simulink model "MdXX_RspToNetWork"  (R2024b)
settings: Solver=FixedStepDiscrete  StartTime=0.0  StopTime=10.0  FixedStep=0.01  RelTol=1e-3
(part 3 of 3)

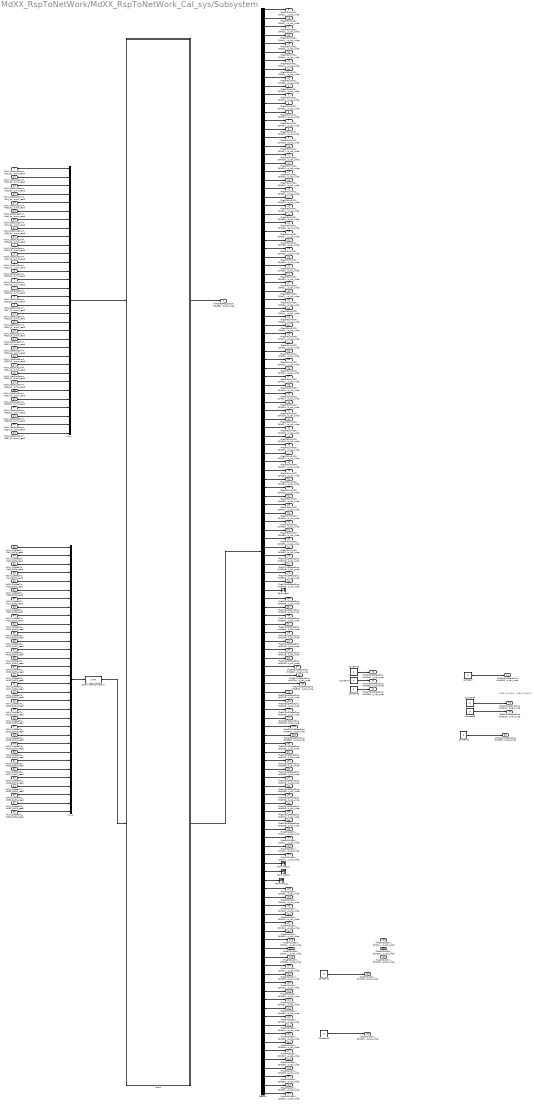
== system MdXX_RspToNetWork/MdXX_RspToNetWork_Cal_sys/Subsystem ==
  note: Md53占用Md18，Md56占用Md25
  MdXX_RspOutComm_Md1_RspOutComm_read : Inport
  MdXX_RspOutComm_Md10_RspOutComm_read : Inport  Port=2
  MdXX_RspOutComm_Md11_RspOutComm_read : Inport  Port=3
  MdXX_RspOutComm_Md12_RspOutComm_read : Inport  Port=4
  MdXX_RspOutComm_Md13_RspOutComm_read : Inport  Port=5
  MdXX_RspOutComm_Md14_RspOutComm_read : Inport  Port=6
  MdXX_RspOutComm_Md15_RspOutComm_read : Inport  Port=7
  MdXX_RspOutComm_Md16_RspOutComm_read : Inport  Port=8
  MdXX_RspOutComm_Md17_RspOutComm_read : Inport  Port=9
  MdXX_RspOutComm_Md18_RspOutComm_read : Inport  Port=10
  MdXX_RspOutComm_Md19_RspOutComm_read : Inport  Port=11
  MdXX_RspOutComm_Md2_RspOutComm_read : Inport  Port=12
  MdXX_RspOutComm_Md20_RspOutComm_read : Inport  Port=13
  MdXX_RspOutComm_Md21_RspOutComm_read : Inport  Port=14
  MdXX_RspOutComm_Md22_RspOutComm_read : Inport  Port=15
  MdXX_RspOutComm_Md23_RspOutComm_read : Inport  Port=16
  MdXX_RspOutComm_Md24_RspOutComm_read : Inport  Port=17
  MdXX_RspOutComm_Md25_RspOutComm_read : Inport  Port=18
  MdXX_RspOutComm_Md26_RspOutComm_read : Inport  Port=19
  MdXX_RspOutComm_Md27_RspOutComm_read : Inport  Port=20
  MdXX_RspOutComm_Md28_RspOutComm_read : Inport  Port=21
  MdXX_RspOutComm_Md29_RspOutComm_read : Inport  Port=22
  MdXX_RspOutComm_Md3_RspOutComm_read : Inport  Port=23
  MdXX_RspOutComm_Md30_RspOutComm_read : Inport  Port=24
  MdXX_RspOutComm_Md31_RspOutComm_read : Inport  Port=25
  MdXX_RspOutComm_Md32_RspOutComm_read : Inport  Port=26
  MdXX_RspOutComm_Md4_RspOutComm_read : Inport  Port=27
  MdXX_RspOutComm_Md5_RspOutComm_read : Inport  Port=28
  MdXX_RspOutComm_Md6_RspOutComm_read : Inport  Port=29
  MdXX_RspOutComm_Md7_RspOutComm_read : Inport  Port=30
  MdXX_RspOutComm_Md8_RspOutComm_read : Inport  Port=31
  MdXX_RspOutComm_Md9_RspOutComm_read : Inport  Port=32
  MdXX_SrcReqTp_Md1_SrcTp_read : Inport  Port=33
  MdXX_SrcReqTp_Md10_SrcTp_read : Inport  Port=34
  MdXX_SrcReqTp_Md11_SrcTp_read : Inport  Port=35
  MdXX_SrcReqTp_Md12_SrcTp_read : Inport  Port=36
  MdXX_SrcReqTp_Md13_SrcTp_read : Inport  Port=37
  MdXX_SrcReqTp_Md14_SrcTp_read : Inport  Port=38
  MdXX_SrcReqTp_Md15_SrcTp_read : Inport  Port=39
  MdXX_SrcReqTp_Md16_SrcTp_read : Inport  Port=40
  MdXX_SrcReqTp_Md17_SrcTp_read : Inport  Port=41
  MdXX_SrcReqTp_Md18_SrcTp_read : Inport  Port=42
  MdXX_SrcReqTp_Md19_SrcTp_read : Inport  Port=43
  MdXX_SrcReqTp_Md2_SrcTp_read : Inport  Port=44
  MdXX_SrcReqTp_Md20_SrcTp_read : Inport  Port=45
  MdXX_SrcReqTp_Md21_SrcTp_read : Inport  Port=46
  MdXX_SrcReqTp_Md22_SrcTp_read : Inport  Port=47
  MdXX_SrcReqTp_Md23_SrcTp_read : Inport  Port=48
  MdXX_SrcReqTp_Md24_SrcTp_read : Inport  Port=49
  MdXX_SrcReqTp_Md25_SrcTp_read : Inport  Port=50
  MdXX_SrcReqTp_Md26_SrcTp_read : Inport  Port=51
  MdXX_SrcReqTp_Md27_SrcTp_read : Inport  Port=52
  MdXX_SrcReqTp_Md28_SrcTp_read : Inport  Port=53
  MdXX_SrcReqTp_Md29_SrcTp_read : Inport  Port=54
  MdXX_SrcReqTp_Md3_SrcTp_read : Inport  Port=55
  MdXX_SrcReqTp_Md30_SrcTp_read : Inport  Port=56
  MdXX_SrcReqTp_Md31_SrcTp_read : Inport  Port=57
  MdXX_SrcReqTp_Md32_SrcTp_read : Inport  Port=58
  MdXX_SrcReqTp_Md4_SrcTp_read : Inport  Port=59
  MdXX_SrcReqTp_Md5_SrcTp_read : Inport  Port=60
  MdXX_SrcReqTp_Md6_SrcTp_read : Inport  Port=61
  MdXX_SrcReqTp_Md7_SrcTp_read : Inport  Port=62
  MdXX_SrcReqTp_Md8_SrcTp_read : Inport  Port=63
  MdXX_SrcReqTp_Md9_SrcTp_read : Inport  Port=64
  Chart : Stateflow chart  TreatAsAtomicUnit=on
  Constant{,1..8} (9 alike) : Constant  Value=0  OutDataTypeStr=uint8
  Data Type Conversion : DataTypeConversion  OutDataTypeStr=uint8  SaturateOnIntegerOverflow=off  RndMeth=Floor
  Demux : Demux  Outputs=128
  Mux : Mux  Inputs=32
  Mux1 : Mux  Inputs=32
  Terminator{,1..3} (4 alike) : Terminator
  IfVeSMStPassCmprtMd_RfCtrl_Sw_RclRspStat_Val_write : Outport  VectorParamsAs1DForOutWhenUnconnected=off
      settings: EnsureOutportIsVirtual=on
  IfVeSMSuHMI2L_StMd1_Rsp_Val_write : Outport  Port=2  VectorParamsAs1DForOutWhenUnconnected=off
      settings: EnsureOutportIsVirtual=on
  IfVeSMSuHMI2L_StMd10_Rsp_Val_write : Outport  Port=3  VectorParamsAs1DForOutWhenUnconnected=off
      settings: EnsureOutportIsVirtual=on
  IfVeSMSuHMI2L_StMd11_Rsp_Val_write : Outport  Port=4  VectorParamsAs1DForOutWhenUnconnected=off
      settings: EnsureOutportIsVirtual=on
  IfVeSMSuHMI2L_StMd12_Rsp_Val_write : Outport  Port=5  VectorParamsAs1DForOutWhenUnconnected=off
      settings: EnsureOutportIsVirtual=on
  IfVeSMSuHMI2L_StMd13_Rsp_Val_write : Outport  Port=6  VectorParamsAs1DForOutWhenUnconnected=off
      settings: EnsureOutportIsVirtual=on
  IfVeSMSuHMI2L_StMd14_Rsp_Val_write : Outport  Port=7  VectorParamsAs1DForOutWhenUnconnected=off
      settings: EnsureOutportIsVirtual=on
  IfVeSMSuHMI2L_StMd15_Rsp_Val_write : Outport  Port=8  VectorParamsAs1DForOutWhenUnconnected=off
      settings: EnsureOutportIsVirtual=on
  IfVeSMSuHMI2L_StMd16_Rsp_Val_write : Outport  Port=9  VectorParamsAs1DForOutWhenUnconnected=off
      settings: EnsureOutportIsVirtual=on
  IfVeSMSuHMI2L_StMd17_Rsp_Val_write : Outport  Port=10  VectorParamsAs1DForOutWhenUnconnected=off
      settings: EnsureOutportIsVirtual=on
  IfVeSMSuHMI2L_StMd18_Rsp_Val_write : Outport  Port=11  VectorParamsAs1DForOutWhenUnconnected=off
      settings: EnsureOutportIsVirtual=on
  IfVeSMSuHMI2L_StMd19_Rsp_Val_write : Outport  Port=12  VectorParamsAs1DForOutWhenUnconnected=off
      settings: EnsureOutportIsVirtual=on
  IfVeSMSuHMI2L_StMd2_Rsp_Val_write : Outport  Port=13  VectorParamsAs1DForOutWhenUnconnected=off
      settings: EnsureOutportIsVirtual=on
  IfVeSMSuHMI2L_StMd20_Rsp_Val_write : Outport  Port=14  VectorParamsAs1DForOutWhenUnconnected=off
      settings: EnsureOutportIsVirtual=on
  IfVeSMSuHMI2L_StMd21_Rsp_Val_write : Outport  Port=15  VectorParamsAs1DForOutWhenUnconnected=off
      settings: EnsureOutportIsVirtual=on
  IfVeSMSuHMI2L_StMd22_Rsp_Val_write : Outport  Port=16  VectorParamsAs1DForOutWhenUnconnected=off
      settings: EnsureOutportIsVirtual=on
  IfVeSMSuHMI2L_StMd23_Rsp_Val_write : Outport  Port=17  VectorParamsAs1DForOutWhenUnconnected=off
      settings: EnsureOutportIsVirtual=on
  IfVeSMSuHMI2L_StMd24_Rsp_Val_write : Outport  Port=18  VectorParamsAs1DForOutWhenUnconnected=off
      settings: EnsureOutportIsVirtual=on
  IfVeSMSuHMI2L_StMd25_Rsp_Val_write : Outport  Port=19  VectorParamsAs1DForOutWhenUnconnected=off
      settings: EnsureOutportIsVirtual=on
  IfVeSMSuHMI2L_StMd26_Rsp_Val_write : Outport  Port=20  VectorParamsAs1DForOutWhenUnconnected=off
      settings: EnsureOutportIsVirtual=on
  IfVeSMSuHMI2L_StMd27_Rsp_Val_write : Outport  Port=21  VectorParamsAs1DForOutWhenUnconnected=off
      settings: EnsureOutportIsVirtual=on
  IfVeSMSuHMI2L_StMd28_Rsp_Val_write : Outport  Port=22  VectorParamsAs1DForOutWhenUnconnected=off
      settings: EnsureOutportIsVirtual=on
  IfVeSMSuHMI2L_StMd29_Rsp_Val_write : Outport  Port=23  VectorParamsAs1DForOutWhenUnconnected=off
      settings: EnsureOutportIsVirtual=on
  IfVeSMSuHMI2L_StMd3_Rsp_Val_write : Outport  Port=24  VectorParamsAs1DForOutWhenUnconnected=off
      settings: EnsureOutportIsVirtual=on
  IfVeSMSuHMI2L_StMd30_Rsp_Val_write : Outport  Port=25  VectorParamsAs1DForOutWhenUnconnected=off
      settings: EnsureOutportIsVirtual=on
  IfVeSMSuHMI2L_StMd31_Rsp_Val_write : Outport  Port=26  VectorParamsAs1DForOutWhenUnconnected=off
      settings: EnsureOutportIsVirtual=on
  IfVeSMSuHMI2L_StMd32_Rsp_Val_write : Outport  Port=27  VectorParamsAs1DForOutWhenUnconnected=off
      settings: EnsureOutportIsVirtual=on
  IfVeSMSuHMI2L_StMd4_Rsp_Val_write : Outport  Port=28  VectorParamsAs1DForOutWhenUnconnected=off
      settings: EnsureOutportIsVirtual=on
  IfVeSMSuHMI2L_StMd5_Rsp_Val_write : Outport  Port=29  VectorParamsAs1DForOutWhenUnconnected=off
      settings: EnsureOutportIsVirtual=on
  IfVeSMSuHMI2L_StMd6_Rsp_Val_write : Outport  Port=30  VectorParamsAs1DForOutWhenUnconnected=off
      settings: EnsureOutportIsVirtual=on
  IfVeSMSuHMI2L_StMd7_Rsp_Val_write : Outport  Port=31  VectorParamsAs1DForOutWhenUnconnected=off
      settings: EnsureOutportIsVirtual=on
  IfVeSMSuHMI2L_StMd8_Rsp_Val_write : Outport  Port=32  VectorParamsAs1DForOutWhenUnconnected=off
      settings: EnsureOutportIsVirtual=on
  IfVeSMSuHMI2L_StMd9_Rsp_Val_write : Outport  Port=33  VectorParamsAs1DForOutWhenUnconnected=off
      settings: EnsureOutportIsVirtual=on
  IfVeSMSuHMI2R_StMd1_Rsp_Val_write : Outport  Port=34  VectorParamsAs1DForOutWhenUnconnected=off
      settings: EnsureOutportIsVirtual=on
  IfVeSMSuHMI2R_StMd10_Rsp_Val_write : Outport  Port=35  VectorParamsAs1DForOutWhenUnconnected=off
      settings: EnsureOutportIsVirtual=on
  IfVeSMSuHMI2R_StMd11_Rsp_Val_write : Outport  Port=36  VectorParamsAs1DForOutWhenUnconnected=off
      settings: EnsureOutportIsVirtual=on
  IfVeSMSuHMI2R_StMd12_Rsp_Val_write : Outport  Port=37  VectorParamsAs1DForOutWhenUnconnected=off
      settings: EnsureOutportIsVirtual=on
  IfVeSMSuHMI2R_StMd13_Rsp_Val_write : Outport  Port=38  VectorParamsAs1DForOutWhenUnconnected=off
      settings: EnsureOutportIsVirtual=on
  IfVeSMSuHMI2R_StMd14_Rsp_Val_write : Outport  Port=39  VectorParamsAs1DForOutWhenUnconnected=off
      settings: EnsureOutportIsVirtual=on
  IfVeSMSuHMI2R_StMd15_Rsp_Val_write : Outport  Port=40  VectorParamsAs1DForOutWhenUnconnected=off
      settings: EnsureOutportIsVirtual=on
  IfVeSMSuHMI2R_StMd16_Rsp_Val_write : Outport  Port=41  VectorParamsAs1DForOutWhenUnconnected=off
      settings: EnsureOutportIsVirtual=on
  IfVeSMSuHMI2R_StMd17_Rsp_Val_write : Outport  Port=42  VectorParamsAs1DForOutWhenUnconnected=off
      settings: EnsureOutportIsVirtual=on
  IfVeSMSuHMI2R_StMd18_Rsp_Val_write : Outport  Port=43  VectorParamsAs1DForOutWhenUnconnected=off
      settings: EnsureOutportIsVirtual=on
  IfVeSMSuHMI2R_StMd19_Rsp_Val_write : Outport  Port=44  VectorParamsAs1DForOutWhenUnconnected=off
      settings: EnsureOutportIsVirtual=on
  IfVeSMSuHMI2R_StMd2_Rsp_Val_write : Outport  Port=45  VectorParamsAs1DForOutWhenUnconnected=off
      settings: EnsureOutportIsVirtual=on
  IfVeSMSuHMI2R_StMd20_Rsp_Val_write : Outport  Port=46  VectorParamsAs1DForOutWhenUnconnected=off
      settings: EnsureOutportIsVirtual=on
  IfVeSMSuHMI2R_StMd21_Rsp_Val_write : Outport  Port=47  VectorParamsAs1DForOutWhenUnconnected=off
      settings: EnsureOutportIsVirtual=on
  IfVeSMSuHMI2R_StMd22_Rsp_Val_write : Outport  Port=48  VectorParamsAs1DForOutWhenUnconnected=off
      settings: EnsureOutportIsVirtual=on
  IfVeSMSuHMI2R_StMd23_Rsp_Val_write : Outport  Port=49  VectorParamsAs1DForOutWhenUnconnected=off
      settings: EnsureOutportIsVirtual=on
  IfVeSMSuHMI2R_StMd24_Rsp_Val_write : Outport  Port=50  VectorParamsAs1DForOutWhenUnconnected=off
      settings: EnsureOutportIsVirtual=on
  IfVeSMSuHMI2R_StMd25_Rsp_Val_write : Outport  Port=51  VectorParamsAs1DForOutWhenUnconnected=off
      settings: EnsureOutportIsVirtual=on
  IfVeSMSuHMI2R_StMd26_Rsp_Val_write : Outport  Port=52  VectorParamsAs1DForOutWhenUnconnected=off
      settings: EnsureOutportIsVirtual=on
  IfVeSMSuHMI2R_StMd27_Rsp_Val_write : Outport  Port=53  VectorParamsAs1DForOutWhenUnconnected=off
      settings: EnsureOutportIsVirtual=on
  IfVeSMSuHMI2R_StMd28_Rsp_Val_write : Outport  Port=54  VectorParamsAs1DForOutWhenUnconnected=off
      settings: EnsureOutportIsVirtual=on
  IfVeSMSuHMI2R_StMd29_Rsp_Val_write : Outport  Port=55  VectorParamsAs1DForOutWhenUnconnected=off
      settings: EnsureOutportIsVirtual=on
  IfVeSMSuHMI2R_StMd3_Rsp_Val_write : Outport  Port=56  VectorParamsAs1DForOutWhenUnconnected=off
      settings: EnsureOutportIsVirtual=on
  IfVeSMSuHMI2R_StMd30_Rsp_Val_write : Outport  Port=57  VectorParamsAs1DForOutWhenUnconnected=off
      settings: EnsureOutportIsVirtual=on
  IfVeSMSuHMI2R_StMd31_Rsp_Val_write : Outport  Port=58  VectorParamsAs1DForOutWhenUnconnected=off
      settings: EnsureOutportIsVirtual=on
  IfVeSMSuHMI2R_StMd32_Rsp_Val_write : Outport  Port=59  VectorParamsAs1DForOutWhenUnconnected=off
      settings: EnsureOutportIsVirtual=on
  IfVeSMSuHMI2R_StMd4_Rsp_Val_write : Outport  Port=60  VectorParamsAs1DForOutWhenUnconnected=off
      settings: EnsureOutportIsVirtual=on
  IfVeSMSuHMI2R_StMd5_Rsp_Val_write : Outport  Port=61  VectorParamsAs1DForOutWhenUnconnected=off
      settings: EnsureOutportIsVirtual=on
  IfVeSMSuHMI2R_StMd6_Rsp_Val_write : Outport  Port=62  VectorParamsAs1DForOutWhenUnconnected=off
      settings: EnsureOutportIsVirtual=on
  IfVeSMSuHMI2R_StMd7_Rsp_Val_write : Outport  Port=63  VectorParamsAs1DForOutWhenUnconnected=off
      settings: EnsureOutportIsVirtual=on
  IfVeSMSuHMI2R_StMd8_Rsp_Val_write : Outport  Port=64  VectorParamsAs1DForOutWhenUnconnected=off
      settings: EnsureOutportIsVirtual=on
  IfVeSMSuHMI2R_StMd9_Rsp_Val_write : Outport  Port=65  VectorParamsAs1DForOutWhenUnconnected=off
      settings: EnsureOutportIsVirtual=on
  IfVeSMSuStPassCmprtMd10RclRspStat_Val_write : Outport  Port=66  VectorParamsAs1DForOutWhenUnconnected=off
      settings: EnsureOutportIsVirtual=on
  IfVeSMSuStPassCmprtMd11RclRspStat_Val_write : Outport  Port=67  VectorParamsAs1DForOutWhenUnconnected=off
      settings: EnsureOutportIsVirtual=on
  IfVeSMSuStPassCmprtMd12RclRspStat_Val_write : Outport  Port=68  VectorParamsAs1DForOutWhenUnconnected=off
      settings: EnsureOutportIsVirtual=on
  IfVeSMSuStPassCmprtMd13RclRspStat_Val_write : Outport  Port=69  VectorParamsAs1DForOutWhenUnconnected=off
      settings: EnsureOutportIsVirtual=on
  IfVeSMSuStPassCmprtMd14RclRspStat_Val_write : Outport  Port=70  VectorParamsAs1DForOutWhenUnconnected=off
      settings: EnsureOutportIsVirtual=on
  IfVeSMSuStPassCmprtMd15RclRspStat_Val_write : Outport  Port=71  VectorParamsAs1DForOutWhenUnconnected=off
      settings: EnsureOutportIsVirtual=on
  IfVeSMSuStPassCmprtMd16RclRspStat_Val_write : Outport  Port=72  VectorParamsAs1DForOutWhenUnconnected=off
      settings: EnsureOutportIsVirtual=on
  IfVeSMSuStPassCmprtMd17RclRspStat_Val_write : Outport  Port=73  VectorParamsAs1DForOutWhenUnconnected=off
      settings: EnsureOutportIsVirtual=on
  IfVeSMSuStPassCmprtMd18RclRspStat_Val_write : Outport  Port=74  VectorParamsAs1DForOutWhenUnconnected=off
      settings: EnsureOutportIsVirtual=on
  IfVeSMSuStPassCmprtMd19RclRspStat_Val_write : Outport  Port=75  VectorParamsAs1DForOutWhenUnconnected=off
      settings: EnsureOutportIsVirtual=on
  IfVeSMSuStPassCmprtMd1RclRspStat_Val_write : Outport  Port=76  VectorParamsAs1DForOutWhenUnconnected=off
      settings: EnsureOutportIsVirtual=on
  IfVeSMSuStPassCmprtMd20RclRspStat_Val_write : Outport  Port=77  VectorParamsAs1DForOutWhenUnconnected=off
      settings: EnsureOutportIsVirtual=on
  IfVeSMSuStPassCmprtMd21RclRspStat_Val_write : Outport  Port=78  VectorParamsAs1DForOutWhenUnconnected=off
      settings: EnsureOutportIsVirtual=on
  IfVeSMSuStPassCmprtMd22RclRspStat_Val_write : Outport  Port=79  VectorParamsAs1DForOutWhenUnconnected=off
      settings: EnsureOutportIsVirtual=on
  IfVeSMSuStPassCmprtMd23RclRspStat_Val_write : Outport  Port=80  VectorParamsAs1DForOutWhenUnconnected=off
      settings: EnsureOutportIsVirtual=on
  IfVeSMSuStPassCmprtMd24RclRspStat_Val_write : Outport  Port=81  VectorParamsAs1DForOutWhenUnconnected=off
      settings: EnsureOutportIsVirtual=on
  IfVeSMSuStPassCmprtMd25RclRspStat_Val_write : Outport  Port=82  VectorParamsAs1DForOutWhenUnconnected=off
      settings: EnsureOutportIsVirtual=on
  IfVeSMSuStPassCmprtMd26RclRspStat_Val_write : Outport  Port=83  VectorParamsAs1DForOutWhenUnconnected=off
      settings: EnsureOutportIsVirtual=on
  IfVeSMSuStPassCmprtMd27RclRspStat_Val_write : Outport  Port=84  VectorParamsAs1DForOutWhenUnconnected=off
      settings: EnsureOutportIsVirtual=on
  IfVeSMSuStPassCmprtMd28RclRspStat_Val_write : Outport  Port=85  VectorParamsAs1DForOutWhenUnconnected=off
      settings: EnsureOutportIsVirtual=on
  IfVeSMSuStPassCmprtMd29RclRspStat_Val_write : Outport  Port=86  VectorParamsAs1DForOutWhenUnconnected=off
      settings: EnsureOutportIsVirtual=on
  IfVeSMSuStPassCmprtMd2RclRspStat_Val_write : Outport  Port=87  VectorParamsAs1DForOutWhenUnconnected=off
      settings: EnsureOutportIsVirtual=on
  IfVeSMSuStPassCmprtMd30RclRspStat_Val_write : Outport  Port=88  VectorParamsAs1DForOutWhenUnconnected=off
      settings: EnsureOutportIsVirtual=on
  IfVeSMSuStPassCmprtMd31RclRspStat_Val_write : Outport  Port=89  VectorParamsAs1DForOutWhenUnconnected=off
      settings: EnsureOutportIsVirtual=on
  IfVeSMSuStPassCmprtMd32RclRspStat_Val_write : Outport  Port=90  VectorParamsAs1DForOutWhenUnconnected=off
      settings: EnsureOutportIsVirtual=on
  IfVeSMSuStPassCmprtMd3RclRspStat_Val_write : Outport  Port=91  VectorParamsAs1DForOutWhenUnconnected=off
      settings: EnsureOutportIsVirtual=on
  IfVeSMSuStPassCmprtMd4RclRspStat_Val_write : Outport  Port=92  VectorParamsAs1DForOutWhenUnconnected=off
      settings: EnsureOutportIsVirtual=on
  IfVeSMSuStPassCmprtMd5RclRspStat_Val_write : Outport  Port=93  VectorParamsAs1DForOutWhenUnconnected=off
      settings: EnsureOutportIsVirtual=on
  IfVeSMSuStPassCmprtMd6RclRspStat_Val_write : Outport  Port=94  VectorParamsAs1DForOutWhenUnconnected=off
      settings: EnsureOutportIsVirtual=on
  IfVeSMSuStPassCmprtMd7RclRspStat_Val_write : Outport  Port=95  VectorParamsAs1DForOutWhenUnconnected=off
      settings: EnsureOutportIsVirtual=on
  IfVeSMSuStPassCmprtMd8RclRspStat_Val_write : Outport  Port=96  VectorParamsAs1DForOutWhenUnconnected=off
      settings: EnsureOutportIsVirtual=on
  IfVeSMSuStPassCmprtMd9RclRspStat_Val_write : Outport  Port=97  VectorParamsAs1DForOutWhenUnconnected=off
      settings: EnsureOutportIsVirtual=on
  IfVeSMSuStSrv_StMd1_Rsp_Val_write : Outport  Port=98  VectorParamsAs1DForOutWhenUnconnected=off
      settings: EnsureOutportIsVirtual=on
  IfVeSMSuStSrv_StMd10_Rsp_Val_write : Outport  Port=99  VectorParamsAs1DForOutWhenUnconnected=off
      settings: EnsureOutportIsVirtual=on
  IfVeSMSuStSrv_StMd11_Rsp_Val_write : Outport  Port=100  VectorParamsAs1DForOutWhenUnconnected=off
      settings: EnsureOutportIsVirtual=on
  IfVeSMSuStSrv_StMd12_Rsp_Val_write : Outport  Port=101  VectorParamsAs1DForOutWhenUnconnected=off
      settings: EnsureOutportIsVirtual=on
  IfVeSMSuStSrv_StMd13_Rsp_Val_write : Outport  Port=102  VectorParamsAs1DForOutWhenUnconnected=off
      settings: EnsureOutportIsVirtual=on
  IfVeSMSuStSrv_StMd14_Rsp_Val_write : Outport  Port=103  VectorParamsAs1DForOutWhenUnconnected=off
      settings: EnsureOutportIsVirtual=on
  IfVeSMSuStSrv_StMd15_Rsp_Val_write : Outport  Port=104  VectorParamsAs1DForOutWhenUnconnected=off
      settings: EnsureOutportIsVirtual=on
  IfVeSMSuStSrv_StMd16_Rsp_Val_write : Outport  Port=105  VectorParamsAs1DForOutWhenUnconnected=off
      settings: EnsureOutportIsVirtual=on
  IfVeSMSuStSrv_StMd17_Rsp_Val_write : Outport  Port=106  VectorParamsAs1DForOutWhenUnconnected=off
      settings: EnsureOutportIsVirtual=on
  IfVeSMSuStSrv_StMd18_Rsp_Val_write : Outport  Port=107  VectorParamsAs1DForOutWhenUnconnected=off
      settings: EnsureOutportIsVirtual=on
  IfVeSMSuStSrv_StMd19_Rsp_Val_write : Outport  Port=108  VectorParamsAs1DForOutWhenUnconnected=off
      settings: EnsureOutportIsVirtual=on
  IfVeSMSuStSrv_StMd2_Rsp_Val_write : Outport  Port=109  VectorParamsAs1DForOutWhenUnconnected=off
      settings: EnsureOutportIsVirtual=on
  IfVeSMSuStSrv_StMd20_Rsp_Val_write : Outport  Port=110  VectorParamsAs1DForOutWhenUnconnected=off
      settings: EnsureOutportIsVirtual=on
  IfVeSMSuStSrv_StMd21_Rsp_Val_write : Outport  Port=111  VectorParamsAs1DForOutWhenUnconnected=off
      settings: EnsureOutportIsVirtual=on
  IfVeSMSuStSrv_StMd22_Rsp_Val_write : Outport  Port=112  VectorParamsAs1DForOutWhenUnconnected=off
      settings: EnsureOutportIsVirtual=on
  IfVeSMSuStSrv_StMd23_Rsp_Val_write : Outport  Port=113  VectorParamsAs1DForOutWhenUnconnected=off
      settings: EnsureOutportIsVirtual=on
  IfVeSMSuStSrv_StMd24_Rsp_Val_write : Outport  Port=114  VectorParamsAs1DForOutWhenUnconnected=off
      settings: EnsureOutportIsVirtual=on
  IfVeSMSuStSrv_StMd25_Rsp_Val_write : Outport  Port=115  VectorParamsAs1DForOutWhenUnconnected=off
      settings: EnsureOutportIsVirtual=on
  IfVeSMSuStSrv_StMd26_Rsp_Val_write : Outport  Port=116  VectorParamsAs1DForOutWhenUnconnected=off
      settings: EnsureOutportIsVirtual=on
  IfVeSMSuStSrv_StMd27_Rsp_Val_write : Outport  Port=117  VectorParamsAs1DForOutWhenUnconnected=off
      settings: EnsureOutportIsVirtual=on
  IfVeSMSuStSrv_StMd28_Rsp_Val_write : Outport  Port=118  VectorParamsAs1DForOutWhenUnconnected=off
      settings: EnsureOutportIsVirtual=on
  IfVeSMSuStSrv_StMd29_Rsp_Val_write : Outport  Port=119  VectorParamsAs1DForOutWhenUnconnected=off
      settings: EnsureOutportIsVirtual=on
  IfVeSMSuStSrv_StMd3_Rsp_Val_write : Outport  Port=120  VectorParamsAs1DForOutWhenUnconnected=off
      settings: EnsureOutportIsVirtual=on
  IfVeSMSuStSrv_StMd30_Rsp_Val_write : Outport  Port=121  VectorParamsAs1DForOutWhenUnconnected=off
      settings: EnsureOutportIsVirtual=on
  IfVeSMSuStSrv_StMd31_Rsp_Val_write : Outport  Port=122  VectorParamsAs1DForOutWhenUnconnected=off
      settings: EnsureOutportIsVirtual=on
  IfVeSMSuStSrv_StMd32_Rsp_Val_write : Outport  Port=123  VectorParamsAs1DForOutWhenUnconnected=off
      settings: EnsureOutportIsVirtual=on
  IfVeSMSuStSrv_StMd4_Rsp_Val_write : Outport  Port=124  VectorParamsAs1DForOutWhenUnconnected=off
      settings: EnsureOutportIsVirtual=on
  IfVeSMSuStSrv_StMd5_Rsp_Val_write : Outport  Port=125  VectorParamsAs1DForOutWhenUnconnected=off
      settings: EnsureOutportIsVirtual=on
  IfVeSMSuStSrv_StMd6_Rsp_Val_write : Outport  Port=126  VectorParamsAs1DForOutWhenUnconnected=off
      settings: EnsureOutportIsVirtual=on
  IfVeSMSuStSrv_StMd7_Rsp_Val_write : Outport  Port=127  VectorParamsAs1DForOutWhenUnconnected=off
      settings: EnsureOutportIsVirtual=on
  IfVeSMSuStSrv_StMd8_Rsp_Val_write : Outport  Port=128  VectorParamsAs1DForOutWhenUnconnected=off
      settings: EnsureOutportIsVirtual=on
  IfVeSMSuStSrv_StMd9_Rsp_Val_write : Outport  Port=129  VectorParamsAs1DForOutWhenUnconnected=off
      settings: EnsureOutportIsVirtual=on
  IfVeSMSuStPassCmprtMd53RclRspStat_Val_write : Outport  Port=130  VectorParamsAs1DForOutWhenUnconnected=off
      settings: EnsureOutportIsVirtual=on
  IfVeSMSuStPassCmprtMd56RclRspStat_Val_write : Outport  Port=131  VectorParamsAs1DForOutWhenUnconnected=off
      settings: EnsureOutportIsVirtual=on
  IfVeSMSuStSrv_StMd53_Rsp_Val_write : Outport  Port=132  VectorParamsAs1DForOutWhenUnconnected=off
      settings: EnsureOutportIsVirtual=on
  IfVeSMSuStSrv_StMd56_Rsp_Val_write : Outport  Port=133  VectorParamsAs1DForOutWhenUnconnected=off
      settings: EnsureOutportIsVirtual=on
  IfVeSMSuStPassCmprtMd57RclRspStat_Val_write : Outport  Port=134  VectorParamsAs1DForOutWhenUnconnected=off
      settings: EnsureOutportIsVirtual=on
  IfVeSMSuStPassCmprtMd58RclRspStat_Val_write : Outport  Port=135  VectorParamsAs1DForOutWhenUnconnected=off
      settings: EnsureOutportIsVirtual=on
  IfVeSMSuStPassCmprtMd61RclRspStat_Val_write : Outport  Port=136  VectorParamsAs1DForOutWhenUnconnected=off
      settings: EnsureOutportIsVirtual=on
  IfVeSMSuStPassCmprtMd62RclRspStat_Val_write : Outport  Port=137  VectorParamsAs1DForOutWhenUnconnected=off
      settings: EnsureOutportIsVirtual=on
  wires:
  MdXX_RspOutComm_Md14_RspOutComm_read/1 -> Mux/14
  MdXX_RspOutComm_Md15_RspOutComm_read/1 -> Mux/15
  MdXX_RspOutComm_Md16_RspOutComm_read/1 -> Mux/16
  MdXX_RspOutComm_Md12_RspOutComm_read/1 -> Mux/12
  MdXX_RspOutComm_Md13_RspOutComm_read/1 -> Mux/13
  MdXX_RspOutComm_Md17_RspOutComm_read/1 -> Mux/17
  MdXX_RspOutComm_Md18_RspOutComm_read/1 -> Mux/18
  MdXX_RspOutComm_Md10_RspOutComm_read/1 -> Mux/10
  MdXX_RspOutComm_Md11_RspOutComm_read/1 -> Mux/11
  MdXX_RspOutComm_Md19_RspOutComm_read/1 -> Mux/19
  MdXX_RspOutComm_Md20_RspOutComm_read/1 -> Mux/20
  MdXX_RspOutComm_Md8_RspOutComm_read/1 -> Mux/8
  MdXX_RspOutComm_Md9_RspOutComm_read/1 -> Mux/9
  MdXX_RspOutComm_Md21_RspOutComm_read/1 -> Mux/21
  MdXX_RspOutComm_Md22_RspOutComm_read/1 -> Mux/22
  MdXX_RspOutComm_Md6_RspOutComm_read/1 -> Mux/6
  MdXX_RspOutComm_Md7_RspOutComm_read/1 -> Mux/7
  MdXX_RspOutComm_Md23_RspOutComm_read/1 -> Mux/23
  MdXX_RspOutComm_Md24_RspOutComm_read/1 -> Mux/24
  MdXX_RspOutComm_Md25_RspOutComm_read/1 -> Mux/25
  MdXX_RspOutComm_Md3_RspOutComm_read/1 -> Mux/3
  MdXX_RspOutComm_Md4_RspOutComm_read/1 -> Mux/4
  MdXX_RspOutComm_Md5_RspOutComm_read/1 -> Mux/5
  MdXX_RspOutComm_Md26_RspOutComm_read/1 -> Mux/26
  MdXX_RspOutComm_Md27_RspOutComm_read/1 -> Mux/27
  MdXX_RspOutComm_Md1_RspOutComm_read/1 -> Mux/1
  MdXX_RspOutComm_Md2_RspOutComm_read/1 -> Mux/2
  MdXX_RspOutComm_Md28_RspOutComm_read/1 -> Mux/28
  MdXX_RspOutComm_Md29_RspOutComm_read/1 -> Mux/29
  MdXX_RspOutComm_Md30_RspOutComm_read/1 -> Mux/30
  MdXX_RspOutComm_Md31_RspOutComm_read/1 -> Mux/31
  MdXX_RspOutComm_Md32_RspOutComm_read/1 -> Mux/32
  Mux/1 -> Chart/1(MdXX_RspOutCommArray)
  MdXX_SrcReqTp_Md10_SrcTp_read/1 -> Mux1/10
  MdXX_SrcReqTp_Md11_SrcTp_read/1 -> Mux1/11
  MdXX_SrcReqTp_Md9_SrcTp_read/1 -> Mux1/9
  MdXX_SrcReqTp_Md12_SrcTp_read/1 -> Mux1/12
  MdXX_SrcReqTp_Md13_SrcTp_read/1 -> Mux1/13
  MdXX_SrcReqTp_Md14_SrcTp_read/1 -> Mux1/14
  MdXX_SrcReqTp_Md6_SrcTp_read/1 -> Mux1/6
  MdXX_SrcReqTp_Md7_SrcTp_read/1 -> Mux1/7
  MdXX_SrcReqTp_Md8_SrcTp_read/1 -> Mux1/8
  MdXX_SrcReqTp_Md15_SrcTp_read/1 -> Mux1/15
  MdXX_SrcReqTp_Md16_SrcTp_read/1 -> Mux1/16
  MdXX_SrcReqTp_Md4_SrcTp_read/1 -> Mux1/4
  MdXX_SrcReqTp_Md5_SrcTp_read/1 -> Mux1/5
  MdXX_SrcReqTp_Md17_SrcTp_read/1 -> Mux1/17
  MdXX_SrcReqTp_Md18_SrcTp_read/1 -> Mux1/18
  MdXX_SrcReqTp_Md19_SrcTp_read/1 -> Mux1/19
  MdXX_SrcReqTp_Md20_SrcTp_read/1 -> Mux1/20
  MdXX_SrcReqTp_Md2_SrcTp_read/1 -> Mux1/2
  MdXX_SrcReqTp_Md3_SrcTp_read/1 -> Mux1/3
  MdXX_SrcReqTp_Md21_SrcTp_read/1 -> Mux1/21
  MdXX_SrcReqTp_Md22_SrcTp_read/1 -> Mux1/22
  MdXX_SrcReqTp_Md23_SrcTp_read/1 -> Mux1/23
  MdXX_SrcReqTp_Md1_SrcTp_read/1 -> Mux1/1
  MdXX_SrcReqTp_Md24_SrcTp_read/1 -> Mux1/24
  MdXX_SrcReqTp_Md25_SrcTp_read/1 -> Mux1/25
  MdXX_SrcReqTp_Md26_SrcTp_read/1 -> Mux1/26
  MdXX_SrcReqTp_Md27_SrcTp_read/1 -> Mux1/27
  MdXX_SrcReqTp_Md28_SrcTp_read/1 -> Mux1/28
  MdXX_SrcReqTp_Md29_SrcTp_read/1 -> Mux1/29
  MdXX_SrcReqTp_Md30_SrcTp_read/1 -> Mux1/30
  MdXX_SrcReqTp_Md31_SrcTp_read/1 -> Mux1/31
  MdXX_SrcReqTp_Md32_SrcTp_read/1 -> Mux1/32
  Mux1/1 -> Data Type Conversion/1
  Data Type Conversion/1 -> Chart/2(MdXX_SrcReqTpArray)
  Chart/1(RfCtrl_Sw_RclRspStat) -> IfVeSMStPassCmprtMd_RfCtrl_Sw_RclRspStat_Val_write/1
  Demux/81 -> IfVeSMSuStPassCmprtMd17RclRspStat_Val_write/1
  Demux/77 -> IfVeSMSuStPassCmprtMd13RclRspStat_Val_write/1
  Demux/83 -> IfVeSMSuStPassCmprtMd19RclRspStat_Val_write/1
  Demux/74 -> IfVeSMSuStPassCmprtMd10RclRspStat_Val_write/1
  Demux/75 -> IfVeSMSuStPassCmprtMd11RclRspStat_Val_write/1
  Demux/76 -> IfVeSMSuStPassCmprtMd12RclRspStat_Val_write/1
  Demux/72 -> IfVeSMSuStPassCmprtMd8RclRspStat_Val_write/1
  Demux/73 -> IfVeSMSuStPassCmprtMd9RclRspStat_Val_write/1
  Demux/84 -> IfVeSMSuStPassCmprtMd20RclRspStat_Val_write/1
  Demux/87 -> IfVeSMSuStPassCmprtMd23RclRspStat_Val_write/1
  Demux/97 -> IfVeSMSuStSrv_StMd1_Rsp_Val_write/1
  Demux/98 -> IfVeSMSuStSrv_StMd2_Rsp_Val_write/1
  Demux/99 -> IfVeSMSuStSrv_StMd3_Rsp_Val_write/1
  Demux/100 -> IfVeSMSuStSrv_StMd4_Rsp_Val_write/1
  Demux/104 -> IfVeSMSuStSrv_StMd8_Rsp_Val_write/1
  Demux/105 -> IfVeSMSuStSrv_StMd9_Rsp_Val_write/1
  Demux/106 -> IfVeSMSuStSrv_StMd10_Rsp_Val_write/1
  Demux/107 -> IfVeSMSuStSrv_StMd11_Rsp_Val_write/1
  Demux/108 -> IfVeSMSuStSrv_StMd12_Rsp_Val_write/1
  Demux/109 -> IfVeSMSuStSrv_StMd13_Rsp_Val_write/1
  Demux/113 -> IfVeSMSuStSrv_StMd17_Rsp_Val_write/1
  Demux/115 -> IfVeSMSuStSrv_StMd19_Rsp_Val_write/1
  Demux/116 -> IfVeSMSuStSrv_StMd20_Rsp_Val_write/1
  Demux/117 -> IfVeSMSuStSrv_StMd21_Rsp_Val_write/1
  Demux/118 -> IfVeSMSuStSrv_StMd22_Rsp_Val_write/1
  Demux/119 -> IfVeSMSuStSrv_StMd23_Rsp_Val_write/1
  Demux/120 -> IfVeSMSuStSrv_StMd24_Rsp_Val_write/1
  Demux/122 -> IfVeSMSuStSrv_StMd26_Rsp_Val_write/1
  Demux/123 -> IfVeSMSuStSrv_StMd27_Rsp_Val_write/1
  Demux/124 -> IfVeSMSuStSrv_StMd28_Rsp_Val_write/1
  Demux/125 -> IfVeSMSuStSrv_StMd29_Rsp_Val_write/1
  Demux/126 -> IfVeSMSuStSrv_StMd30_Rsp_Val_write/1
  Demux/127 -> IfVeSMSuStSrv_StMd31_Rsp_Val_write/1
  Demux/128 -> IfVeSMSuStSrv_StMd32_Rsp_Val_write/1
  Demux/66 -> IfVeSMSuStPassCmprtMd2RclRspStat_Val_write/1
  Demux/67 -> IfVeSMSuStPassCmprtMd3RclRspStat_Val_write/1
  Demux/68 -> IfVeSMSuStPassCmprtMd4RclRspStat_Val_write/1
  Demux/88 -> IfVeSMSuStPassCmprtMd24RclRspStat_Val_write/1
  Demux/90 -> IfVeSMSuStPassCmprtMd26RclRspStat_Val_write/1
  Demux/91 -> IfVeSMSuStPassCmprtMd27RclRspStat_Val_write/1
  Demux/92 -> IfVeSMSuStPassCmprtMd28RclRspStat_Val_write/1
  Demux/65 -> IfVeSMSuStPassCmprtMd1RclRspStat_Val_write/1
  Demux/93 -> IfVeSMSuStPassCmprtMd29RclRspStat_Val_write/1
  Demux/64 -> IfVeSMSuHMI2R_StMd32_Rsp_Val_write/1
  Demux/94 -> IfVeSMSuStPassCmprtMd30RclRspStat_Val_write/1
  Demux/62 -> IfVeSMSuHMI2R_StMd30_Rsp_Val_write/1
  Demux/63 -> IfVeSMSuHMI2R_StMd31_Rsp_Val_write/1
  Demux/95 -> IfVeSMSuStPassCmprtMd31RclRspStat_Val_write/1
  Demux/96 -> IfVeSMSuStPassCmprtMd32RclRspStat_Val_write/1
  Demux/60 -> IfVeSMSuHMI2R_StMd28_Rsp_Val_write/1
  Demux/61 -> IfVeSMSuHMI2R_StMd29_Rsp_Val_write/1
  Demux/57 -> IfVeSMSuHMI2R_StMd25_Rsp_Val_write/1
  Demux/58 -> IfVeSMSuHMI2R_StMd26_Rsp_Val_write/1
  Demux/59 -> IfVeSMSuHMI2R_StMd27_Rsp_Val_write/1
  Demux/55 -> IfVeSMSuHMI2R_StMd23_Rsp_Val_write/1
  Demux/56 -> IfVeSMSuHMI2R_StMd24_Rsp_Val_write/1
  Demux/51 -> IfVeSMSuHMI2R_StMd19_Rsp_Val_write/1
  Demux/52 -> IfVeSMSuHMI2R_StMd20_Rsp_Val_write/1
  Demux/53 -> IfVeSMSuHMI2R_StMd21_Rsp_Val_write/1
  Demux/54 -> IfVeSMSuHMI2R_StMd22_Rsp_Val_write/1
  Demux/48 -> IfVeSMSuHMI2R_StMd16_Rsp_Val_write/1
  Demux/49 -> IfVeSMSuHMI2R_StMd17_Rsp_Val_write/1
  Demux/50 -> IfVeSMSuHMI2R_StMd18_Rsp_Val_write/1
  Demux/46 -> IfVeSMSuHMI2R_StMd14_Rsp_Val_write/1
  Demux/47 -> IfVeSMSuHMI2R_StMd15_Rsp_Val_write/1
  Demux/43 -> IfVeSMSuHMI2R_StMd11_Rsp_Val_write/1
  Demux/44 -> IfVeSMSuHMI2R_StMd12_Rsp_Val_write/1
  Demux/45 -> IfVeSMSuHMI2R_StMd13_Rsp_Val_write/1
  Demux/42 -> IfVeSMSuHMI2R_StMd10_Rsp_Val_write/1
  Demux/40 -> IfVeSMSuHMI2R_StMd8_Rsp_Val_write/1
  Demux/41 -> IfVeSMSuHMI2R_StMd9_Rsp_Val_write/1
  Demux/37 -> IfVeSMSuHMI2R_StMd5_Rsp_Val_write/1
  Demux/38 -> IfVeSMSuHMI2R_StMd6_Rsp_Val_write/1
  Demux/39 -> IfVeSMSuHMI2R_StMd7_Rsp_Val_write/1
  Demux/35 -> IfVeSMSuHMI2R_StMd3_Rsp_Val_write/1
  Demux/36 -> IfVeSMSuHMI2R_StMd4_Rsp_Val_write/1
  Demux/31 -> IfVeSMSuHMI2L_StMd31_Rsp_Val_write/1
  Demux/32 -> IfVeSMSuHMI2L_StMd32_Rsp_Val_write/1
  Demux/33 -> IfVeSMSuHMI2R_StMd1_Rsp_Val_write/1
  Demux/34 -> IfVeSMSuHMI2R_StMd2_Rsp_Val_write/1
  Demux/27 -> IfVeSMSuHMI2L_StMd27_Rsp_Val_write/1
  Demux/28 -> IfVeSMSuHMI2L_StMd28_Rsp_Val_write/1
  Demux/29 -> IfVeSMSuHMI2L_StMd29_Rsp_Val_write/1
  Demux/30 -> IfVeSMSuHMI2L_StMd30_Rsp_Val_write/1
  Demux/25 -> IfVeSMSuHMI2L_StMd25_Rsp_Val_write/1
  Demux/26 -> IfVeSMSuHMI2L_StMd26_Rsp_Val_write/1
  Demux/22 -> IfVeSMSuHMI2L_StMd22_Rsp_Val_write/1
  Demux/23 -> IfVeSMSuHMI2L_StMd23_Rsp_Val_write/1
  Demux/24 -> IfVeSMSuHMI2L_StMd24_Rsp_Val_write/1
  Demux/21 -> IfVeSMSuHMI2L_StMd21_Rsp_Val_write/1
  Demux/18 -> IfVeSMSuHMI2L_StMd18_Rsp_Val_write/1
  Demux/19 -> IfVeSMSuHMI2L_StMd19_Rsp_Val_write/1
  Demux/20 -> IfVeSMSuHMI2L_StMd20_Rsp_Val_write/1
  Demux/16 -> IfVeSMSuHMI2L_StMd16_Rsp_Val_write/1
  Demux/17 -> IfVeSMSuHMI2L_StMd17_Rsp_Val_write/1
  Demux/13 -> IfVeSMSuHMI2L_StMd13_Rsp_Val_write/1
  Demux/14 -> IfVeSMSuHMI2L_StMd14_Rsp_Val_write/1
  Demux/15 -> IfVeSMSuHMI2L_StMd15_Rsp_Val_write/1
  Demux/11 -> IfVeSMSuHMI2L_StMd11_Rsp_Val_write/1
  Demux/12 -> IfVeSMSuHMI2L_StMd12_Rsp_Val_write/1
  Demux/10 -> IfVeSMSuHMI2L_StMd10_Rsp_Val_write/1
  Demux/7 -> IfVeSMSuHMI2L_StMd7_Rsp_Val_write/1
  Demux/8 -> IfVeSMSuHMI2L_StMd8_Rsp_Val_write/1
  Demux/9 -> IfVeSMSuHMI2L_StMd9_Rsp_Val_write/1
  Demux/5 -> IfVeSMSuHMI2L_StMd5_Rsp_Val_write/1
  Demux/6 -> IfVeSMSuHMI2L_StMd6_Rsp_Val_write/1
  Demux/1 -> IfVeSMSuHMI2L_StMd1_Rsp_Val_write/1
  Demux/2 -> IfVeSMSuHMI2L_StMd2_Rsp_Val_write/1
  Demux/3 -> IfVeSMSuHMI2L_StMd3_Rsp_Val_write/1
  Demux/4 -> IfVeSMSuHMI2L_StMd4_Rsp_Val_write/1
  Chart/2(RspArray) -> Demux/1
  Demux/82 -> IfVeSMSuStPassCmprtMd53RclRspStat_Val_write/1
  Constant/1 -> IfVeSMSuStPassCmprtMd18RclRspStat_Val_write/1
  Demux/89 -> IfVeSMSuStPassCmprtMd56RclRspStat_Val_write/1
  Constant1/1 -> IfVeSMSuStPassCmprtMd25RclRspStat_Val_write/1
  Demux/114 -> IfVeSMSuStSrv_StMd53_Rsp_Val_write/1
  Demux/121 -> IfVeSMSuStSrv_StMd56_Rsp_Val_write/1
  Constant2/1 -> IfVeSMSuStSrv_StMd18_Rsp_Val_write/1
  Constant3/1 -> IfVeSMSuStSrv_StMd25_Rsp_Val_write/1
  Demux/85 -> IfVeSMSuStPassCmprtMd57RclRspStat_Val_write/1
  Demux/86 -> IfVeSMSuStPassCmprtMd58RclRspStat_Val_write/1
  Constant5/1 -> IfVeSMSuStPassCmprtMd22RclRspStat_Val_write/1
  Constant4/1 -> IfVeSMSuStPassCmprtMd21RclRspStat_Val_write/1
  Demux/70 -> IfVeSMSuStPassCmprtMd61RclRspStat_Val_write/1
  Demux/71 -> IfVeSMSuStPassCmprtMd62RclRspStat_Val_write/1
  Demux/69 -> Terminator/1
  Constant6/1 -> IfVeSMSuStPassCmprtMd14RclRspStat_Val_write/1
  Constant7/1 -> IfVeSMSuStPassCmprtMd15RclRspStat_Val_write/1
  Constant8/1 -> IfVeSMSuStPassCmprtMd16RclRspStat_Val_write/1
  Demux/101 -> Terminator1/1
  Demux/102 -> Terminator2/1
  Demux/103 -> Terminator3/1
  Demux/110 -> IfVeSMSuStSrv_StMd6_Rsp_Val_write/1
  Demux/111 -> IfVeSMSuStSrv_StMd7_Rsp_Val_write/1
  Demux/112 -> IfVeSMSuStSrv_StMd5_Rsp_Val_write/1
  Demux/78 -> IfVeSMSuStPassCmprtMd6RclRspStat_Val_write/1
  Demux/79 -> IfVeSMSuStPassCmprtMd7RclRspStat_Val_write/1
  Demux/80 -> IfVeSMSuStPassCmprtMd5RclRspStat_Val_write/1

== stateflow chart MdXX_RspToNetWork/MdXX_RspToNetWork_Cal_sys/Subsystem/Chart ==
  (default) -> (junction 7)
  (junction 7) -> (junction 9) : {
      | i=0;
      | RspArray = 0;
      | }
  (junction 11) -> (junction 13) [order 1] : [MdXX_SrcReqTpArray[i]>1 &&MdXX_SrcReqTpArray[i]<6]
  (junction 9) -> (junction 11) [order 1] : [i<32]
  (junction 11) -> (junction 15) [order 2]
  (junction 13) -> (junction 20) : {
      | index = (MdXX_SrcReqTpArray[i]-2)*32+i;
      | RspArray[index] =MdXX_RspOutCommArray[i];
      | }
  (junction 15) -> (junction 9) : {i=i+1;}
  (junction 9) -> (junction 18) [order 2] : {
      | i=0;
      | RfCtrl_Sw_RclRspStat = 0;
      | }
  (junction 20) -> (junction 15)
  (junction 31) -> (junction 33) [order 1] : [MdXX_SrcReqTpArray[i]==6&&MdXX_RspOutCommArray[i]!=0]
  (junction 18) -> (junction 31) [order 1] : [i<32]
  (junction 31) -> (junction 35) [order 2]
  (junction 33) -> (junction 39) : {RfCtrl_Sw_RclRspStat = MdXX_RspOutCommArray[i];}
  (junction 35) -> (junction 18) : {i=i+1;}
  (junction 18) -> (junction 41) [order 2]
  (junction 39) -> (junction 41)
  data: RfCtrl_Sw_RclRspStat output uint8; MdXX_RspOutCommArray input size=32; MdXX_SrcReqTpArray input size=32; RspArray output uint8 size=128; i local uint8; index local uint8
